simulink model "contract_test"  (R2017a)
settings: Solver=FixedStepDiscrete  StartTime=0.0  StopTime=10.0  FixedStep=1  RelTol=1e-3
libraries: Kind x2
settings Model: Creator=mudat  LastModifiedBy=mudat

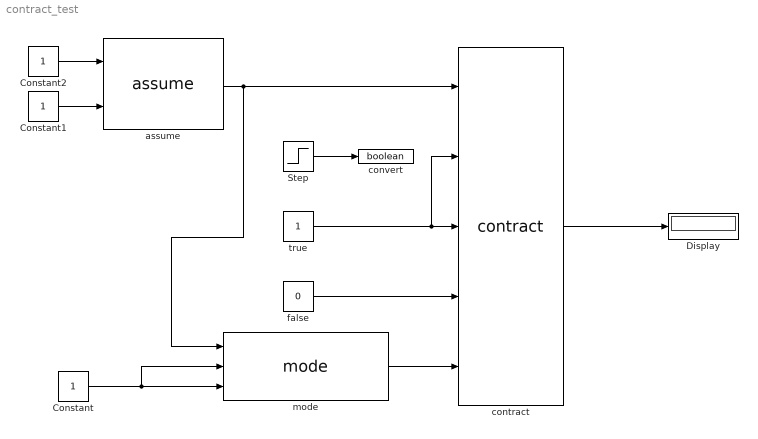
== system contract_test ==
  Constant : Constant  OutDataTypeStr=boolean
  Constant1 : Constant  OutDataTypeStr=boolean
  Constant2 : Constant  OutDataTypeStr=boolean
  Display : Display
  Step : Step  SampleTime=0
  assume : Kind/assume
  contract : M-S-Function  FunctionName=contract  mask{assumePorts=2, guaranteePorts=2, modePorts=1}
      mask prompts: assumePorts "Assume ports     :"; guaranteePorts "Guarantee ports :"; modePorts "Mode ports        :"
      mask init:
      | set_param(gcb,'LinkStatus','none');
      mask Callback assumePorts: contract_callback('inputs_callback',gcb)
      mask Callback guaranteePorts: contract_callback('inputs_callback',gcb)
      mask Callback modePorts: contract_callback('inputs_callback',gcb)
      mask Display:
      | port_label('input',1,'assume')
      | port_label('input',2,'assume')
      | port_label('input',3,'guarantee')
      | port_label('input',4,'guarantee')
      | port_label('input',5,'mode')
      | port_label('output',1,'valid')
  convert : DataTypeConversion  OutDataTypeStr=boolean
  false : Constant  Value=0  OutDataTypeStr=boolean
  mode : Kind/mode
  true : Constant  OutDataTypeStr=boolean
  wires:
  false/1 -> contract/4
  Step/1 -> convert/1
  true/1 -> contract/2, contract/3
  contract/1 -> Display/1
  Constant1/1 -> assume/2
  Constant2/1 -> assume/1
  assume/1 -> mode/1, contract/1
  mode/1 -> contract/5
  Constant/1 -> mode/2, mode/3
